simulink model "DMC_AltSpeedController"  (Simulink 7.4)
settings: Solver=ode1  StartTime=0.0  StopTime=100  FixedStep=Ts  RelTol=1e-3
values from neighbouring files (symbols this model uses):
  I2 = zeros(m,n)    [matricesDMC.m]
  M = (A'*alfa*A+lambda)\A'*alfa    [matricesDMC.m]
  m = t+n    [matricesDMC.m]
  n = length(Su)    [matricesDMC.m]
  P = modelo_quadrotor.solido.m*modelo_quadrotor.solido.g    [modelo.m]
  Q1 = zeros(n,n)    [matricesDMC.m]
  Saux = [Su; ones(m-n,1)*Su(end)]    [matricesDMC.m]
  Su = Su(2:end)    [matricesDMC.m]
  Ts = 0.1    [matricesDMC.m]    (also in modelo.m)
  Vreferencia = 1    [modelo.m]
libraries: quadrotor_models_lineal x1
settings Model: Creator=g28115dq  LastModifiedBy=g28115dq

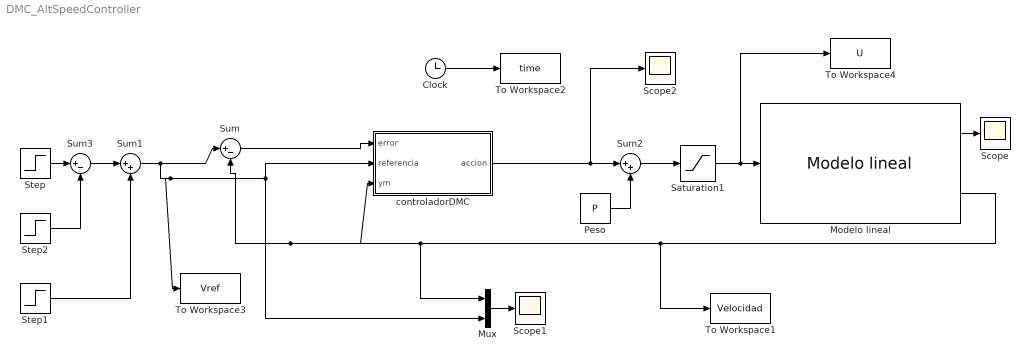
== system DMC_AltSpeedController ==
  Clock : Clock
      settings: Decimation=10
  Modelo lineal : quadrotor_models_lineal/Modelo lineal  SystemSampleTime=-1
  Mux : Mux  Inputs=2
  Peso : Constant  Value=P  OutDataType=fixdt(1, 16)  OutScaling=2^0
  Saturation1 : Saturate  UpperLimit=32  LowerLimit=0  SampleTime=Ts  OutDataType=fixdt(1, 16)  OutScaling=2^0
  Scope : Scope
  Scope1 : Scope
      settings: TimeRange=30  YMin=-1.05  YMax=-0.95
  Scope2 : Scope
      settings: SaveName=ScopeData2
  Step : Step  Time=50  After=Vreferencia  SampleTime=0
  Step1 : Step  Time=65  After=Vreferencia*0.5  SampleTime=0
  Step2 : Step  Time=80  After=Vreferencia*2.5  SampleTime=0
  Sum : Sum  Inputs=|+-  OutDataType=fixdt(1, 16)  OutScaling=2^0
  Sum1 : Sum  Inputs=|++  OutDataType=fixdt(1, 16)  OutScaling=2^0
  Sum2 : Sum  Inputs=|++  OutDataType=fixdt(1, 16)  OutScaling=2^0
  Sum3 : Sum  Inputs=|+-  OutDataType=fixdt(1, 16)  OutScaling=2^0
  To Workspace1 : ToWorkspace  VariableName=Velocidad  SampleTime=-1  SaveFormat=Array
  To Workspace2 : ToWorkspace  VariableName=time  SampleTime=-1  SaveFormat=Array
  To Workspace3 : ToWorkspace  VariableName=Vref  SampleTime=-1  SaveFormat=Array
  To Workspace4 : ToWorkspace  VariableName=U  SampleTime=-1  SaveFormat=Array
  controladorDMC : Subsystem
  wires:
  Sum1/1 -> Sum/1, To Workspace3/1, Mux/2, controladorDMC/2(referencia)
  Sum/1 -> controladorDMC/1(error)
  Modelo lineal/2 -> Mux/1, Sum/2, controladorDMC/3(ym), To Workspace1/1
  Modelo lineal/1 -> Scope/1
  Mux/1 -> Scope1/1
  Clock/1 -> To Workspace2/1
  Step1/1 -> Sum1/2
  Peso/1 -> Sum2/2
  Sum2/1 -> Saturation1/1
  Sum3/1 -> Sum1/1
  Step/1 -> Sum3/1
  Step2/1 -> Sum3/2
  Saturation1/1 -> To Workspace4/1, Modelo lineal/1
  controladorDMC/1(accion) -> Sum2/1, Scope2/1

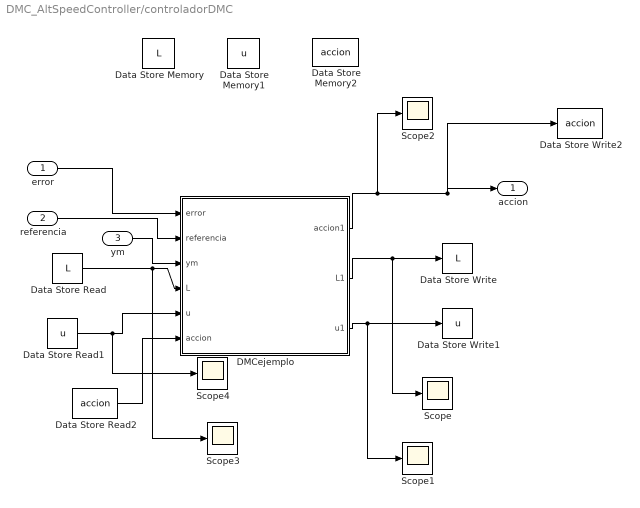
== system DMC_AltSpeedController/controladorDMC ==
  error : Inport
  referencia : Inport  Port=2
  ym : Inport  Port=3
  DMCejemplo : Stateflow chart
  Data Store Memory : DataStoreMemory  DataStoreName=L  InitialValue=zeros(n,1)  OutDataType=fixdt(1, 16)  OutScaling=2^0
  Data Store Memory1 : DataStoreMemory  DataStoreName=u  InitialValue=zeros(t,1)  OutDataType=fixdt(1, 16)  OutScaling=2^0
  Data Store Memory2 : DataStoreMemory  DataStoreName=accion  OutDataType=fixdt(1, 16)  OutScaling=2^0
  Data Store Read : DataStoreRead  DataStoreName=L  SampleTime=0
  Data Store Read1 : DataStoreRead  DataStoreName=u  SampleTime=0
  Data Store Read2 : DataStoreRead  DataStoreName=accion  SampleTime=0
  Data Store Write : DataStoreWrite  DataStoreName=L  SampleTime=-1
  Data Store Write1 : DataStoreWrite  DataStoreName=u  SampleTime=-1
  Data Store Write2 : DataStoreWrite  DataStoreName=accion  SampleTime=-1
  Scope{,1..4} (5 alike) : Scope
      Scope settings: SaveName=ScopeData5
      Scope1 settings: TimeRange=0.2390468870099923  YMin=-0.08774509803921574  YMax=0.8926470588235292  SaveName=ScopeData6
      Scope2 settings: SaveName=ScopeData7
      Scope3 settings: SaveName=ScopeData8
      Scope4 settings: TimeRange=0.2390468870099923  YMin=-0.08774509803921574  YMax=0.8926470588235292  SaveName=ScopeData9
  accion : Outport
  wires:
  DMCejemplo/3(u1) -> Data Store Write1/1, Scope1/1
  DMCejemplo/2(L1) -> Data Store Write/1, Scope/1
  DMCejemplo/1(accion1) -> Scope2/1, Data Store Write2/1, accion/1
  error/1 -> DMCejemplo/1(error)
  referencia/1 -> DMCejemplo/2(referencia)
  Data Store Read/1 -> DMCejemplo/4(L), Scope3/1
  Data Store Read1/1 -> DMCejemplo/5(u), Scope4/1
  Data Store Read2/1 -> DMCejemplo/6(accion)
  ym/1 -> DMCejemplo/3(ym)

== matlab function controladorDMC/DMCejemplo ==
  data: accion1 output double; error input double; referencia input double; ym input double; L input double; u input double; accion input double; L1 output double; u1 output double; m parameter double; Q1 parameter double; Su parameter double; I2 parameter double; M parameter double; Saux parameter double
function [accion1,L1,u1] = DMCejemplo(error,referencia,ym,L,u,accion,m,Q1,Su,I2,M,Saux)
%#eml

command_upper_limit= 3.3;
command_lower_limit=-3.3;
y=referencia-error;
r=referencia; %referencia
R=Saux;

%R=r*ones(m,1);%vector de trayectoria de referencia  //esto no funciona
for i=1:m
    R(i)=r;
end
L1=Q1*L+Su*u(1); %Actualizo la respuesta libre
w=Saux;
for i=1:m
   w(i)=ym-L1(1);
end
%w=Saux*0;
%w=(y-L(1))*ones(m,1); %perturbacion no medible  //el ones(m,1) no funciona en simulink
N=I2*L1+w;
D=R-N;
u1=M*D;

accion1=accion+u1(1);  %Aplico la accion de control

if accion1>command_upper_limit
    accion1 = command_upper_limit;
    u1(1)   = accion1 - accion;
end
if accion1<command_lower_limit
    accion1 = command_lower_limit;
    u1(1)   = accion1 - accion;
end

end
